simulink model "attack_kin_controller_eightpath_ROS"  (R2020b)
settings: Solver=ode8  StartTime=0.0  StopTime=inf  FixedStep=Ts  RelTol=1e-3
values from neighbouring files (symbols this model uses):
  BDD_thresh = 1    [Run_model.m]
  d = 0.0562    [Run_model.m]
  I_single = [3;4]    [Run_model.m]
  kx = 1    [Run_model.m]
  ky = 1    [Run_model.m]
  L = 0.235/2    (= 0.1175)    [Run_model.m]
  max_iter = 2000    [Run_model.m]
  n_meas = 6    [Run_model.m]
  nominal_error_range = 0.1    [Run_model.m]
  r = 2    [Run_model.m]
  R_meas = 1e-4    (= 0.0001)    [Run_model.m]
  rw = 0.05    [Run_model.m]
  T_start_attack = .5*T_final    (= 50)    [Run_model.m]
  Ts = 0.03    [Run_model.m]
  u0 = zeros(n_int,1)    [Run_model.m]
  y0 = 0    [Run_model.m]
  z_hat0 = z_initial    [Run_model.m]
  z_initial = [theta0;x0;y0]    [Run_model.m]
undefined symbols (not defined in the file or in its folder): Angular, Linear
libraries: robotlib x8, simulink x5, sharedTrackingLibrary x2, dspsigops x1
settings Model: Creator=sridhar  LastModifiedBy=sridhar

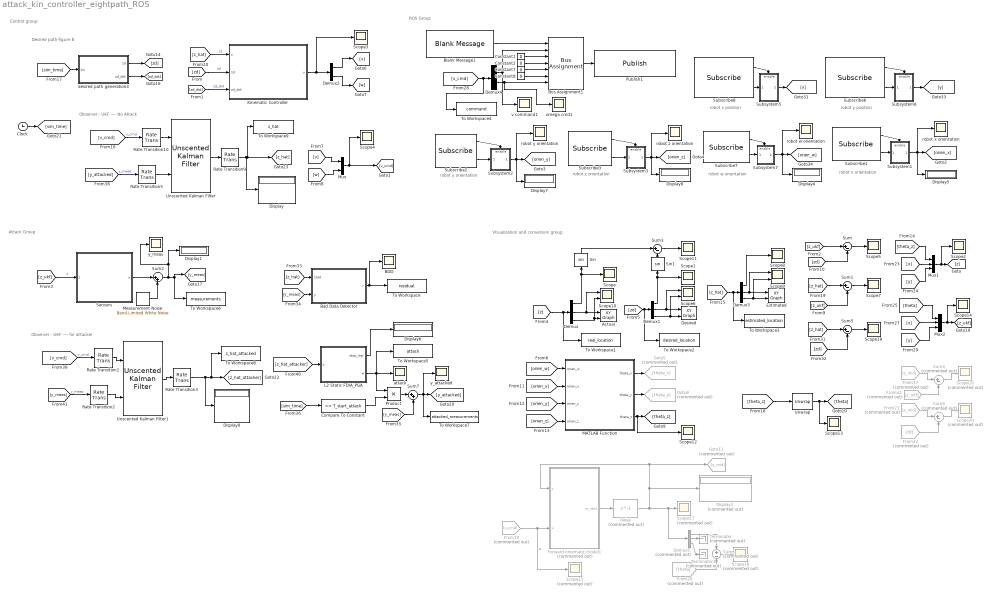
== system attack_kin_controller_eightpath_ROS ==
  note: VIsualization and conversion group
  note: ROS Group
  note: Attack Group
  note: Control group
  note: robot y position
  note: robot x position
  note: robot w orientation
  note: robot x orientation
  note: robot y orientation
  note: robot z orientation
  note: Observer - UKF ---- No Attack
  note: Observer - UKF ---- for attacker
  note: Desired path-figure 8
  " robot w orientation" : Scope
  " robot x orientation" : Scope
  " robot y orientation" : Scope
  " robot z orientation" : Scope
  Actual : simulink/Sinks/XY Graph  xmin=-2  xmax=2  ymin=-1  ymax=1  st=-1
  BDD : Scope
  Bad Data Detector : MATLAB Function  TreatAsAtomicUnit=on
  Blank Message1 : robotlib/Blank Message  messageClass=Message  entityType=geometry_msgs/Twist  messageType=geometry_msgs/Twist  SampleTime=-1  legacyBusStruct=off
  Bus Assignment1 : BusAssignment  AssignedSignals=Linear.X,Linear.Y,Linear.Z,Angular.X,Angular.Y,Angular.Z
  Clock : Clock
      settings: Decimation=100
  Compare To Constant : simulink/Logic and Bit Operations/Compare To Constant  relop=>=  const=T_start_attack  OutDataTypeStr=boolean
  Constant{1..2,7..8} (4 alike) : Constant  Value=0
  Delay : Delay  Commented=on  DelayLength=1  InitialCondition=z_initial  UseCircularBuffer=on
  Demux : Demux  Outputs=3
  Demux1 : Demux  Outputs=3
  Demux2 : Demux  Outputs=2
  Demux3 : Demux  Outputs=3
  Demux4 : Demux  Outputs=2
  Demux5 : Demux  Commented=on  Outputs=3
  Desired : simulink/Sinks/XY Graph  xmin=-2  xmax=2  ymin=-1  ymax=1  st=-1
  Display{,1,4..9} (8 alike) : Display
  Display3 : Display  Commented=on
  Estimated : simulink/Sinks/XY Graph  xmin=-2  xmax=2  ymin=-1  ymax=1  st=-1
  Forward kinematic model1 : MATLAB Function  Commented=on  TreatAsAtomicUnit=on
  From21 : From  Commented=on  GotoTag=z_mid
  From22 : From  Commented=on  GotoTag=zd
  From26 : From  Commented=on  GotoTag=theta
  From30 : From  Commented=on  GotoTag=v_cmd
  From37 : From  Commented=on  GotoTag=z_mid
  From42 : From  Commented=on  GotoTag=z_ukf
  Goto11 : Goto  Commented=on  GotoTag=z_mid
  Goto5 : Goto  Commented=on  GotoTag=theta_x
  Goto8 : Goto  Commented=on  GotoTag=theta_y
  Kinematic Controller : MATLAB Function  TreatAsAtomicUnit=on
  L2 Static FDIA_PGA : MATLAB Function  TreatAsAtomicUnit=on
  MATLAB Function : MATLAB Function  TreatAsAtomicUnit=on
  Measurement Noise : simulink/Sources/Band-Limited White Noise  Cov=R_meas*Ts  Ts=Ts  seed=[23341]
  Mux : Mux  Inputs=2
  Mux1 : Mux  Inputs=3
  Mux2 : Mux  Inputs=3
  Product : Product
  Publish1 : robotlib/Publish  topicSource=Specify your own  topic=/mobile_base/commands/velocity  messageType=geometry_msgs/Twist  legacyBusStruct=off  messageQueueLength=1
  Rate Transition1 : RateTransition  InitialCondition=u0  OutPortSampleTime=Ts
  Rate Transition10 : RateTransition  InitialCondition=u0  OutPortSampleTime=Ts
  Rate Transition2 : RateTransition  InitialCondition=y0  OutPortSampleTime=Ts
  Rate Transition3 : RateTransition  InitialCondition=z_hat0  OutPortSampleTime=0
  Rate Transition5 : RateTransition  InitialCondition=y0  OutPortSampleTime=Ts
  Rate Transition9 : RateTransition  InitialCondition=z_hat0  OutPortSampleTime=0
  Scope{,1..5,7..8,11..14,19} (13 alike) : Scope
  Scope10 : Scope  NumInputPorts=2
  Scope{15..18,20} (5 alike) : Scope  Commented=on
  Scope6 : Scope  NumInputPorts=2
  Scope9 : Scope  NumInputPorts=2
  Sensors : MATLAB Function  TreatAsAtomicUnit=on
  Sin : Trigonometry
  Sin1 : Trigonometry
  Subscribe{1..3,6..8} (6 alike) : robotlib/Subscribe  Priority=15  topicSource=Specify your own  topic=/odom  messageType=nav_msgs/Odometry  SampleTime=-1  legacyBusStruct=off  messageQueueLength=1
  Subsystem1 : Subsystem  Priority=16
  Subsystem2 : Subsystem  Priority=16
  Subsystem3 : Subsystem  Priority=16
  Subsystem5 : Subsystem  Priority=16
  Subsystem6 : Subsystem  Priority=16
  Subsystem7 : Subsystem  Priority=16
  Sum{,1,3,5} (4 alike) : Sum  Inputs=|+-
  Sum2 : Sum  Inputs=|++
  Sum4 : Sum  Commented=on  Inputs=|+-
  Sum6 : Sum  Commented=on  Inputs=+-
  Sum7 : Sum  Inputs=|++
  Sum9 : Sum  Commented=on  Inputs=|+-
  Terminator : Terminator  Commented=on
  Terminator1 : Terminator  Commented=on
  To Workspace : ToWorkspace  VariableName=residual  SaveFormat=Timeseries  SampleTime=-1
  To Workspace1 : ToWorkspace  VariableName=real_location  SaveFormat=Timeseries  SampleTime=-1
  To Workspace2 : ToWorkspace  VariableName=desired_location  SaveFormat=Timeseries  SampleTime=-1
  To Workspace3 : ToWorkspace  VariableName=estimated_location  SaveFormat=Timeseries  SampleTime=-1
  To Workspace4 : ToWorkspace  VariableName=command  SaveFormat=Timeseries  SampleTime=-1
  To Workspace5 : ToWorkspace  VariableName=attack  SaveFormat=Timeseries  SampleTime=-1
  To Workspace6 : ToWorkspace  VariableName=measurements  SaveFormat=Timeseries  SampleTime=-1
  To Workspace7 : ToWorkspace  VariableName=attacked_measurements  SaveFormat=Timeseries  SampleTime=-1
  To Workspace8 : ToWorkspace  VariableName=z_hat_attacked  SaveFormat=Timeseries  SampleTime=-1
  To Workspace9 : ToWorkspace  VariableName=z_hat  SaveFormat=Timeseries  SampleTime=-1
  Unscented Kalman Filter : sharedTrackingLibrary/Unscented Kalman Filter  StateTransitionFcn=Dynamicfcn  HasAdditiveProcessNoise=Additive  ProcessNoise=P_diag  HasTimeVaryingProcessNoise=off  HasStateTransitionFcnExtraArgument=1  InitialState=z_hat0  InitialStateCovariance=1  Alpha=1e-3  Beta=2  Kappa=0  MeasurementFcn1=measurement_model  HasMeasurementEnablePort1=off  HasAdditiveMeasurementNoise1=Additive  MeasurementNoise1=R_diag  HasTimeVaryingMeasurementNoise1=off  HasMeasurementFcnExtraArgument1=0  MeasurementFcn2=myMeasurementFcn  HasMeasurementEnablePort2=off  HasAdditiveMeasurementNoise2=Additive  MeasurementNoise2=1  HasTimeVaryingMeasurementNoise2=off  HasMeasurementFcnExtraArgument2=0  MeasurementFcn3=myMeasurementFcn  HasMeasurementEnablePort3=off  HasAdditiveMeasurementNoise3=Additive  MeasurementNoise3=1  HasTimeVaryingMeasurementNoise3=off  HasMeasurementFcnExtraArgument3=0  MeasurementFcn4=myMeasurementFcn  HasMeasurementEnablePort4=off  HasAdditiveMeasurementNoise4=Additive  MeasurementNoise4=1  HasTimeVaryingMeasurementNoise4=off  HasMeasurementFcnExtraArgument4=0  MeasurementFcn5=myMeasurementFcn  HasMeasurementEnablePort5=off  HasAdditiveMeasurementNoise5=Additive  MeasurementNoise5=1  HasTimeVaryingMeasurementNoise5=off  HasMeasurementFcnExtraArgument5=0  EnableMultirate=off  StateTransitionFcnSampleTime=1  MeasurementFcn1SampleTime=1  MeasurementFcn2SampleTime=1  MeasurementFcn3SampleTime=1  MeasurementFcn4SampleTime=1  MeasurementFcn5SampleTime=1  UseCurrentEstimator=on  OutputStateCovariance=off  DataType=double  SampleTime=Ts  NumberOfMeasurements=1
      settings: SourceProductBaseCode=CT,DR,TF,ID,LP,NV,AR,RO,RR,UV,VE
  Unscented Kalman Filter1 : sharedTrackingLibrary/Unscented Kalman Filter  StateTransitionFcn=Dynamicfcn  HasAdditiveProcessNoise=Additive  ProcessNoise=P_diag  HasTimeVaryingProcessNoise=off  HasStateTransitionFcnExtraArgument=1  InitialState=z_hat0  InitialStateCovariance=1  Alpha=1e-2  Beta=2  Kappa=0  MeasurementFcn1=measurement_model  HasMeasurementEnablePort1=off  HasAdditiveMeasurementNoise1=Additive  MeasurementNoise1=R_diag  HasTimeVaryingMeasurementNoise1=off  HasMeasurementFcnExtraArgument1=0  MeasurementFcn2=myMeasurementFcn  HasMeasurementEnablePort2=off  HasAdditiveMeasurementNoise2=Additive  MeasurementNoise2=1  HasTimeVaryingMeasurementNoise2=off  HasMeasurementFcnExtraArgument2=0  MeasurementFcn3=myMeasurementFcn  HasMeasurementEnablePort3=off  HasAdditiveMeasurementNoise3=Additive  MeasurementNoise3=1  HasTimeVaryingMeasurementNoise3=off  HasMeasurementFcnExtraArgument3=0  MeasurementFcn4=myMeasurementFcn  HasMeasurementEnablePort4=off  HasAdditiveMeasurementNoise4=Additive  MeasurementNoise4=1  HasTimeVaryingMeasurementNoise4=off  HasMeasurementFcnExtraArgument4=0  MeasurementFcn5=myMeasurementFcn  HasMeasurementEnablePort5=off  HasAdditiveMeasurementNoise5=Additive  MeasurementNoise5=1  HasTimeVaryingMeasurementNoise5=off  HasMeasurementFcnExtraArgument5=0  EnableMultirate=off  StateTransitionFcnSampleTime=1  MeasurementFcn1SampleTime=1  MeasurementFcn2SampleTime=1  MeasurementFcn3SampleTime=1  MeasurementFcn4SampleTime=1  MeasurementFcn5SampleTime=1  UseCurrentEstimator=on  OutputStateCovariance=off  DataType=double  SampleTime=Ts  NumberOfMeasurements=1
      settings: SourceProductBaseCode=CT,DR,TF,ID,LP,NV,AR,RO,RR,UV,VE
  Unwrap : dspsigops/Unwrap  tol=pi  InputProcessing=Columns as channels (frame based)  running=off
  attack : Scope
  desired path generation4 : MATLAB Function  TreatAsAtomicUnit=on
  omega cmd1 : Scope
  v command1 : Scope
  y_attacked : Scope
  y_meas : Scope
  wires:
  Kinematic Controller/1(u) -> Demux2/1, Scope3/1
  [zd_dot] -> Kinematic Controller/3(zd_dot)  "zd_dot"
  [zd] -> Kinematic Controller/2(zd)  "zd"
  [w] -> Mux/2
  Sum/1 -> Scope5/1
  [zd] -> Sum/2
  [z_ukf] -> Sum/1
  Demux/3 -> Scope10/2, Actual/2
  Demux/2 -> Scope10/1, Actual/1
  Demux/1 -> Sin/1, Scope/1
  [z] -> To Workspace1/1, Demux/1
  Demux1/1 -> Scope1/1, Sin1/1
  [zd] -> To Workspace2/1, Demux1/1
  Demux1/3 -> Desired/2, Scope6/2
  Demux1/2 -> Desired/1, Scope6/1
  Demux4/2 -> Bus Assignment1/7, omega cmd1/1
  Blank Message1/1 -> Bus Assignment1/1
  Constant1/1 -> Bus Assignment1/3
  Constant2/1 -> Bus Assignment1/4
  Constant7/1 -> Bus Assignment1/5
  Constant8/1 -> Bus Assignment1/6
  Bus Assignment1/1 -> Publish1/1
  Demux4/1 -> Bus Assignment1/2, v command1/1
  [v_cmd] -> To Workspace4/1, Demux4/1
  [y] -> Mux1/3
  [x] -> Mux1/2
  Mux1/1 -> Scope2/1, [z]
  Subscribe8/2 -> Subsystem5/1(In1)
  Subscribe8/1 -> Subsystem5/Enable
  Subsystem7/1(<w>) -> Display4/1, " robot w orientation"/1, [orien_w]
  Subsystem5/1(<X>) -> [x]
  Subsystem6/1(<Y>) -> [y]
  Subscribe7/2 -> Subsystem7/1(In1)
  Subscribe7/1 -> Subsystem7/Enable
  Subscribe6/1 -> Subsystem6/Enable
  Subscribe6/2 -> Subsystem6/1(In1)
  Subscribe1/1 -> Subsystem1/Enable
  Subscribe1/2 -> Subsystem1/1(In1)
  Subsystem1/1(<x>) -> Display5/1, [orien_x], " robot x orientation"/1
  Subsystem2/1(<y>) -> " robot y orientation"/1, [orien_y], Display7/1
  Subscribe2/2 -> Subsystem2/1(In1)
  Subscribe2/1 -> Subsystem2/Enable
  Subscribe3/1 -> Subsystem3/Enable
  Subscribe3/2 -> Subsystem3/1(In1)
  Subsystem3/1(<Z>) -> " robot z orientation"/1, Display8/1, [orien_z]
  [orien_w] -> MATLAB Function/1(orien_w)
  [orien_x] -> MATLAB Function/2(orien_x)
  [orien_y] -> MATLAB Function/3(orien_y)
  [orien_z] -> MATLAB Function/4(orien_z)
  MATLAB Function/1(theta_x) -> Goto5/1
  MATLAB Function/2(theta_y) -> Goto8/1
  MATLAB Function/3(theta_z) -> Scope12/1, [theta_z]
  [theta_z] -> Mux1/1
  [z_hat] -> Kinematic Controller/1(z)  "z1"
  [v] -> Mux/1
  Demux2/1 -> [v]
  Demux2/2 -> [w]
  [y_attacked] -> Rate Transition5/1  "y_meas"
  Rate Transition10/1 -> Unscented Kalman Filter/1
  Rate Transition5/1 -> Unscented Kalman Filter/2
  [v_cmd] -> Rate Transition10/1  "v_cmd"
  Rate Transition9/1 -> [z_hat], To Workspace9/1, Display/1
  Unscented Kalman Filter/1 -> Rate Transition9/1
  Sensors/1(y) -> Sum2/1
  Measurement Noise/1 -> Sum2/2
  [z_ukf] -> Sensors/1(z)  "z"
  Demux3/2 -> Scope9/1, Estimated/1
  Demux3/3 -> Scope9/2, Estimated/2
  [z_hat] -> Demux3/1, To Workspace3/1
  Demux3/1 -> Scope8/1
  [z_hat] -> Sum1/1
  [z_ukf] -> Sum1/2
  Sum1/1 -> Scope7/1
  Sin/1 -> Sum3/1
  Sin1/1 -> Sum3/2
  Sum3/1 -> Scope11/1
  [theta] -> Mux2/1
  Mux2/1 -> [z_ukf], Scope14/1
  [x] -> Mux2/2
  [y] -> Mux2/3
  Sum5/1 -> Scope19/1
  [z_hat] -> Sum5/1
  [zd] -> Sum5/2
  [y_meas] -> Bad Data Detector/2(y)
  [z_hat] -> Bad Data Detector/1(zhat)
  Bad Data Detector/1(r) -> To Workspace/1, BDD/1
  Sum2/1 -> Display1/1, y_meas/1, To Workspace6/1, [y_meas]
  [sim_time] -> Compare To Constant/1
  Sum7/1 -> To Workspace7/1, [y_attacked], y_attacked/1
  L2 Static FDIA_PGA/2(e) -> To Workspace5/1, attack/1, Product/1
  [y_meas] -> Sum7/2
  Compare To Constant/1 -> Product/2
  Product/1 -> Sum7/1
  Clock/1 -> [sim_time]
  L2 Static FDIA_PGA/1(stop_iter) -> Display6/1
  [y_meas] -> Rate Transition2/1  "y_meas"
  Rate Transition3/1 -> To Workspace8/1, [z_hat_attacker], Display9/1
  Rate Transition2/1 -> Unscented Kalman Filter1/2
  Unscented Kalman Filter1/1 -> Rate Transition3/1
  Rate Transition1/1 -> Unscented Kalman Filter1/1
  [v_cmd] -> Rate Transition1/1  "v_cmd"
  [z_hat_attacker] -> L2 Static FDIA_PGA/1(z)
  desired path generation4/2(zd_dot) -> [zd_dot]
  desired path generation4/1(zd) -> [zd]
  [sim_time] -> desired path generation4/1(tin)
  [theta_z] -> Unwrap/1
  Unwrap/1 -> Scope13/1, [theta]
  From37/1 -> Sum4/1
  From42/1 -> Sum4/2
  Sum4/1 -> Scope16/1
  From26/1 -> Sum6/2
  Demux5/1 -> Sum6/1
  From30/1 -> Scope15/1, Forward kinematic model1/2(u)  "u"
  Delay/1 -> Demux5/1, Scope17/1, Goto11/1, Forward kinematic model1/1(z), Display3/1
  Sum6/1 -> Scope18/1
  Demux5/2 -> Terminator/1
  Demux5/3 -> Terminator1/1
  Forward kinematic model1/1(zr_next) -> Delay/1
  Mux/1 -> [v_cmd], Scope4/1
  Sum9/1 -> Scope20/1
  From21/1 -> Sum9/1
  From22/1 -> Sum9/2

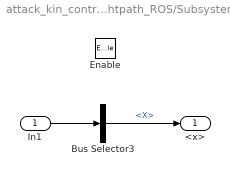
== system attack_kin_controller_eightpath_ROS/Subsystem1 ==
  In1 : Inport
  Enable : EnablePort
  Bus Selector3 : BusSelector  OutputSignals=Pose.Pose.Orientation.X
  <x> : Outport
  wires:
  Bus Selector3/1 -> <x>/1  "<X>"
  In1/1 -> Bus Selector3/1

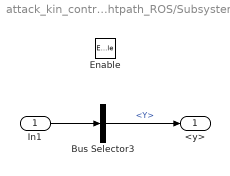
== system attack_kin_controller_eightpath_ROS/Subsystem2 ==
  In1 : Inport
  Enable : EnablePort
  Bus Selector3 : BusSelector  OutputSignals=Pose.Pose.Orientation.Y
  <y> : Outport
  wires:
  In1/1 -> Bus Selector3/1
  Bus Selector3/1 -> <y>/1  "<Y>"

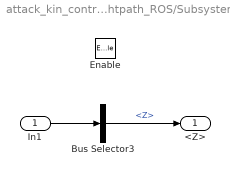
== system attack_kin_controller_eightpath_ROS/Subsystem3 ==
  In1 : Inport
  Enable : EnablePort
  Bus Selector3 : BusSelector  OutputSignals=Pose.Pose.Orientation.Z
  <Z> : Outport
  wires:
  Bus Selector3/1 -> <Z>/1  "<Z>"
  In1/1 -> Bus Selector3/1

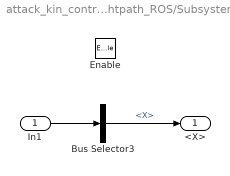
== system attack_kin_controller_eightpath_ROS/Subsystem5 ==
  In1 : Inport
  Enable : EnablePort
  Bus Selector3 : BusSelector  OutputSignals=Pose.Pose.Position.X
  <X> : Outport
  wires:
  In1/1 -> Bus Selector3/1
  Bus Selector3/1 -> <X>/1  "<X>"

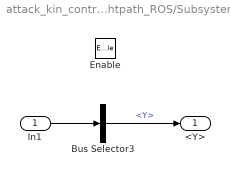
== system attack_kin_controller_eightpath_ROS/Subsystem6 ==
  In1 : Inport
  Enable : EnablePort
  Bus Selector3 : BusSelector  OutputSignals=Pose.Pose.Position.Y
  <Y> : Outport
  wires:
  In1/1 -> Bus Selector3/1
  Bus Selector3/1 -> <Y>/1  "<Y>"

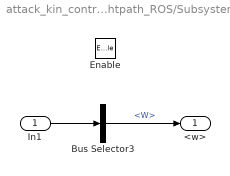
== system attack_kin_controller_eightpath_ROS/Subsystem7 ==
  In1 : Inport
  Enable : EnablePort
  Bus Selector3 : BusSelector  OutputSignals=Pose.Pose.Orientation.W
  <w> : Outport
  wires:
  In1/1 -> Bus Selector3/1
  Bus Selector3/1 -> <w>/1  "<W>"

== matlab function attack_kin_controller_eightpath_ROS/MATLAB Function ==
  data: orien_w input; orien_x input; theta_x output; theta_y output; orien_y input; orien_z input; theta_z output
function [theta_x, theta_y, theta_z] = fcn(orien_w, orien_x, orien_y, orien_z)
% input is [w x y z] 
% output is [z y x]

quat = [orien_w, orien_x, orien_y, orien_z];
eul = quat2eul(quat);

theta_x = eul(3);
theta_y = eul(2);
theta_z = eul(1);

== matlab function attack_kin_controller_eightpath_ROS/Kinematic Controller ==
  data: z input; u output; zd input; zd_dot input; d parameter; kx parameter; ky parameter; r parameter
function u = fcn(z,zd,zd_dot,d, kx, ky, r)

theta = z(1);
x = z(2);
y = z(3);
thetad = zd(1);
xd = zd(2);
yd = zd(3);
thetad_dot = zd_dot(1);
xd_dot = zd_dot(2);
yd_dot = zd_dot(3);

K1 = [cos(theta) sin(theta);
     -sin(theta)/d cos(theta)/d];
K2 = [xd_dot + kx*sin( atan( kx*(xd-x) ) );
      yd_dot + ky*sin( atan( ky*(yd-y) ) )];
  
%   K2 = [xd_dot + kx*cos( atan( kx*(xd-x) ) );
%       yd_dot + ky*sin( atan( ky*(yd-y) ) )];
u = K1*K2;

% v = (xd_dot + kx*sin( atan( kx*(xd-x) ) ))*(cos(theta)) + (yd_dot + ky*sin( atan( ky*(yd-y) ) ))*(sin(theta));
% 
% 
% u = [v; v/r];

== matlab function attack_kin_controller_eightpath_ROS/Sensors ==
  data: z input; y output; n_meas parameter
function y = fcn(z,n_meas)

coder.extrinsic('measurement_model');

y = zeros(n_meas,1);
y(:) = measurement_model(z);

== matlab function attack_kin_controller_eightpath_ROS/Forward kinematic model1 ==
  data: z input; u input; zr_next output; d parameter; Ts parameter
function zr_next = fcn(z,u,d,Ts)

%% unpacking the state vectors
theta=z(1);

%% unpacking the intput
v=u(1);
omega=u(2);

%% ODE
theta_dot=omega;
x_dot=v*cos(theta)-d*omega*sin(theta);
y_dot=v*sin(theta)+d*omega*cos(theta);
% phir_dot = (v+omega)/r;
% phil_dot = (v-omega)/r;


%% packing the output
zr_dot=[theta_dot;x_dot;y_dot];

zr_next = z + Ts*zr_dot;

== matlab function attack_kin_controller_eightpath_ROS/Bad Data Detector ==
  data: zhat input; y input; r output; n_meas parameter; nominal_error_range parameter
function r = fcn(zhat, y,n_meas,nominal_error_range)

coder.extrinsic('measurement_model');

yhat = zeros(n_meas,1);
yhat(:) = measurement_model(zhat);

r = norm(y-yhat,2)-nominal_error_range;

== matlab function attack_kin_controller_eightpath_ROS/L2 Static FDIA_PGA ==
  data: z input; stop_iter output; I_single parameter; e output; BDD_thresh parameter; max_iter parameter; n_meas parameter; rw parameter; L parameter
function [stop_iter,e]  = fcn(z,I_single,BDD_thresh,max_iter, n_meas,rw, L)

coder.extrinsic('L2_FDIA2');
%% Measurement Channel Attack
%  Assumptions:
%  1. The attacker knows the actual measurement
%  2. The attacker can only corrupt upto n_attack measurements
%  3. The attacker knows the BDD theshold

attack_idx = I_single;

C = @(x,y,theta) [-x*sin(theta) cos(theta) 0;
                   y*cos(theta) 0 sin(theta);
                   0 1 0;
                   0 0 1;
                   0 1/(4*rw) L/(4*rw);
                   0 1/(4*rw) -L/(4*rw)];
Cd = C(z(2), z(3), z(1));


e = zeros(n_meas,1);
stop_iter = 0;
[stop_iter(:),e(:)] = L2_FDIA2(Cd,attack_idx,0.6*BDD_thresh,max_iter);

== matlab function attack_kin_controller_eightpath_ROS/desired path generation4 ==
  data: tin input; zd output; zd_dot output; r parameter
function [zd,zd_dot] = fcn(tin,r)

t = tin;
theta_d = t/4;
wd = 1/4;
a=r;

x = a*cos(theta_d)/(1+sin(theta_d)^2);
y = a*sin(theta_d)*cos(theta_d)/(1+sin(theta_d)^2);
% unit circle (radius = 1; origin: (0,0))
zd = [atan(y./x);              % theta
      a*cos(theta_d)/(1+sin(theta_d)^2);         % x
      a*sin(theta_d)*cos(theta_d)/(1+sin(theta_d)^2)];        % y

zd_dot = [wd*cos(theta_d)/(1+sin(theta_d)^2);
          -a*wd*sin(theta_d)*(cos(theta_d)^2+2)/(1+sin(theta_d)^2)^2;
          (a*wd*cos(theta_d)^2-2*a*wd*sin(theta_d)^2)/(1+sin(theta_d)^2)^2];

% z1 = (a*sin(theta_d)^2*cos(theta_d)^3-11*a*cos(theta_d)^3+8*a*cos(theta_d))/(1+sin(theta_d)^2)^3;
% z2 = -2*a*sin(theta_d)*cos(theta_d)*(3+2*cos(theta_d)^2-sin(theta_d)^2)/(1+sin(theta_d)^2)^3;
% zd_ddot = [z1;
%            z2];
